simulink model "inv_180_R"  (R2018a)
settings: Solver=VariableStepAuto  StartTime=0.0  StopTime=0.5  RelTol=1e-3
libraries: powerlib x15, powerlib_meascontrol x3
settings Model: Creator=KUNAL  LastModifiedBy=KUNAL

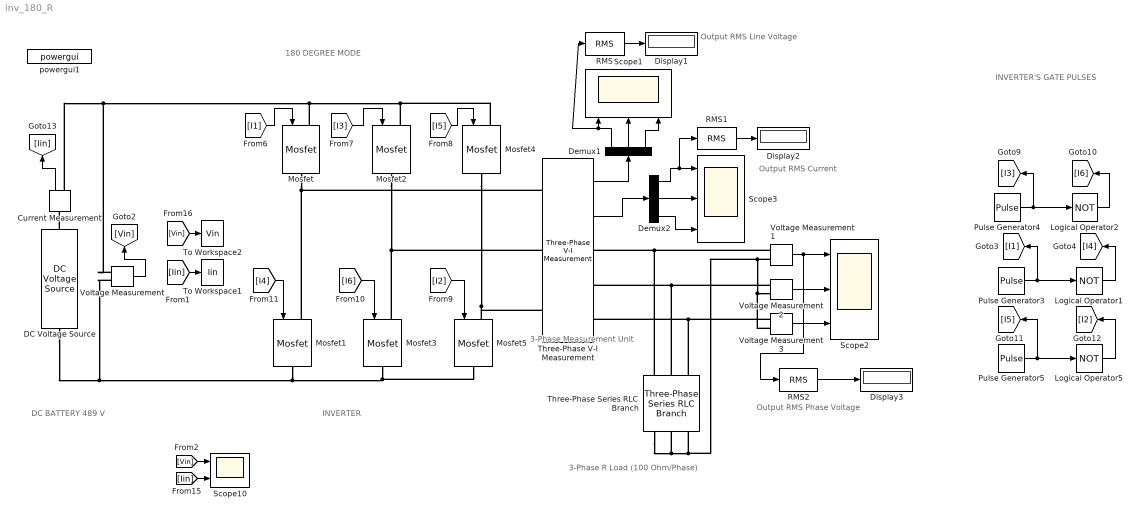
== system inv_180_R ==
  note: INVERTER
  note: INVERTER'S
      | GATE
      | PULSES
  note: 180 DEGREE MODE
  note: DC BATTERY
      | 489 V
  note: Output RMS Current
  note: Output RMS Line Voltage
  note: Output RMS Phase Voltage
  note: 3-Phase Measurement Unit
  note: 3-Phase R Load (100 Ohm/Phase)
  Current Measurement : powerlib/Measurements/Current Measurement  PhasorSimulation=off  OutputType=Complex  PSBequivalent=0
  DC Voltage Source : powerlib/Electrical Sources/DC Voltage Source  Amplitude=489  Measurements=None
  Demux1 : Demux  Outputs=3
  Demux2 : Demux  Outputs=3
  Display1 : Display
  Display2 : Display
  Display3 : Display
  Logical Operator1 : Logic  Operator=NOT  AllPortsSameDT=off  OutDataTypeStr=boolean
  Logical Operator2 : Logic  Operator=NOT  AllPortsSameDT=off  OutDataTypeStr=boolean
  Logical Operator5 : Logic  Operator=NOT  AllPortsSameDT=off  OutDataTypeStr=boolean
  Mosfet{,1..5} (6 alike) : powerlib/Power Electronics/Mosfet  Ron=0  Lon=0  Rd=0  Vfd=0  IC=0  Rs=inf  Cs=0  Measurements=off
  Pulse Generator3 : DiscretePulseGenerator  PulseType=Time based  Period=0.02  PulseWidth=50
  Pulse Generator4 : DiscretePulseGenerator  PulseType=Time based  Period=0.02  PulseWidth=50  PhaseDelay=(120*0.02)/360
  Pulse Generator5 : DiscretePulseGenerator  PulseType=Time based  Period=0.02  PulseWidth=50  PhaseDelay=(240*0.02)/360
  RMS : powerlib_meascontrol/Measurements/RMS  TrueRMS=on  Freq=50  RMSInit=0  Ts=0
  RMS1 : powerlib_meascontrol/Measurements/RMS  TrueRMS=on  Freq=50  RMSInit=0  Ts=0
  RMS2 : powerlib_meascontrol/Measurements/RMS  TrueRMS=on  Freq=50  RMSInit=0  Ts=0
  Scope1 : Scope  NumInputPorts=3
  Scope10 : Scope  NumInputPorts=2
  Scope2 : Scope  NumInputPorts=3
  Scope3 : Scope  NumInputPorts=3
  Three-Phase Series RLC Branch : powerlib/Elements/Three-Phase Series RLC Branch  LConnTagsString=A|B|C  RConnTagsString=A|B|C  BranchType=R  Resistance=10  Inductance=0  Capacitance=0  Measurements=Branch voltages
  Three-Phase V-I Measurement : powerlib/Measurements/Three-Phase V-I Measurement  VoltageMeasurement=phase-to-phase  SetLabelV=off  LabelV=Vabc  Vpu=off  VpuLL=off  CurrentMeasurement=yes  SetLabelI=off  LabelI=Iabc  Ipu=off  Pbase=100e6  Vbase=500e3  OutputType=Complex  PhasorSimulation=off  PSBequivalent=0
  To Workspace1 : ToWorkspace  VariableName=Iin  SaveFormat=Timeseries  SampleTime=-1
  To Workspace2 : ToWorkspace  VariableName=Vin  SaveFormat=Timeseries  SampleTime=-1
  Voltage Measurement{,1..3} (4 alike) : powerlib/Measurements/Voltage Measurement  PhasorSimulation=off  OutputType=Complex  PSBequivalent=0
  powergui1 : powerlib/powergui  Priority=1  SimulationMode=Continuous  SampleTime=50e-6  frequency=60  Iterations=50  frequencyindice=0  Pbase=100e6  ErrMax=1e-4  UnitsV=kV  UnitsW=MW  buscounter=0  FunctionMessages=off  echomessages=off  EnableUseOfTLC=off  CurrentSourceSwitches=off  DisableSnubberDevices=off  DisableRonSwitches=off  DisableVfSwitches=off  DisplayEquations=off  SolverType=Tustin/Backward Euler (TBE)  Interpol=off  ExternalGateDelay=off  methode=off  Ts=100  x0status=blocks  SPID=off  SwTol=0  HookPort=off  RestoreLinks=warning  ResistiveCurrentMeasurement=off  Frange=[0:2:500]  Ylog=off  Xlog=on  ShowGrid=off  save=off  variable=ZData  structure=ScopeData  ZoomFFT=off  StartTime=0.0  cycles=1  DisplayStyle=1  fundamental=60  FreqAxis=off  MaxFrequency=1000  frequencyindicesteady=1  RmsSteady=1  display=off
  wires:
  Pulse Generator3/1 -> [I1], Logical Operator1/1
  Pulse Generator5/1 -> [I5], Logical Operator5/1
  Logical Operator1/1 -> [I4]
  Logical Operator2/1 -> [I6]
  Logical Operator5/1 -> [I2]
  Pulse Generator4/1 -> [I3], Logical Operator2/1
  [I1] -> Mosfet/1
  [I3] -> Mosfet2/1
  [I5] -> Mosfet4/1
  [I2] -> Mosfet5/1
  [I6] -> Mosfet3/1
  [I4] -> Mosfet1/1
  Current Measurement/1 -> [Iin]
  [Vin] -> To Workspace2/1
  [Iin] -> To Workspace1/1
  Voltage Measurement/1 -> [Vin]
  Voltage Measurement3/1 -> Scope2/3
  Demux1/2 -> Scope1/2
  Demux2/3 -> Scope3/3
  Demux2/1 -> Scope3/1, RMS1/1
  Demux1/1 -> Scope1/1, RMS/1
  Three-Phase V-I Measurement/1 -> Demux1/1
  Demux1/3 -> Scope1/3
  Voltage Measurement2/1 -> Scope2/2
  Voltage Measurement1/1 -> Scope2/1, RMS2/1
  Three-Phase V-I Measurement/2 -> Demux2/1
  RMS/1 -> Display1/1
  RMS1/1 -> Display2/1
  Demux2/2 -> Scope3/2
  RMS2/1 -> Display3/1
  [Iin] -> Scope10/2
  [Vin] -> Scope10/1
  connections:
  DC Voltage Source/LConn1 -- Voltage Measurement/LConn2 -- Mosfet1/RConn1 -- Mosfet3/RConn1 -- Mosfet5/RConn1
  Voltage Measurement/LConn1 -- Current Measurement/RConn1 -- Mosfet4/LConn1 -- Mosfet2/LConn1 -- Mosfet/LConn1
  Mosfet/RConn1 -- Three-Phase V-I Measurement/LConn1 -- Mosfet1/LConn1
  Mosfet3/LConn1 -- Three-Phase V-I Measurement/LConn2 -- Mosfet2/RConn1
  Mosfet5/LConn1 -- Three-Phase V-I Measurement/LConn3 -- Mosfet4/RConn1
  DC Voltage Source/RConn1 -- Current Measurement/LConn1
  Voltage Measurement2/LConn2 -- Voltage Measurement3/LConn2 -- Voltage Measurement1/LConn2 -- Three-Phase Series RLC Branch/LConn1 -- Three-Phase Series RLC Branch/LConn2 -- Three-Phase Series RLC Branch/LConn3
  Three-Phase Series RLC Branch/RConn3 -- Three-Phase V-I Measurement/RConn3 -- Voltage Measurement3/LConn1
  Three-Phase Series RLC Branch/RConn1 -- Three-Phase V-I Measurement/RConn1 -- Voltage Measurement1/LConn1
  Three-Phase Series RLC Branch/RConn2 -- Three-Phase V-I Measurement/RConn2 -- Voltage Measurement2/LConn1
